simulink model "DCMotorControl"  (R2014a)
settings: Solver=ode45  StartTime=0.0  StopTime=10.0  RelTol=1e-3
InitFcn:
  | R = 8.70
  | Kt = 0.0334
  | Ke = 0.0334
  | J = 1.80e-6
  | L = 0
  | b = 0
settings Model: Creator=usmankhan  LastModifiedBy=usmankhan

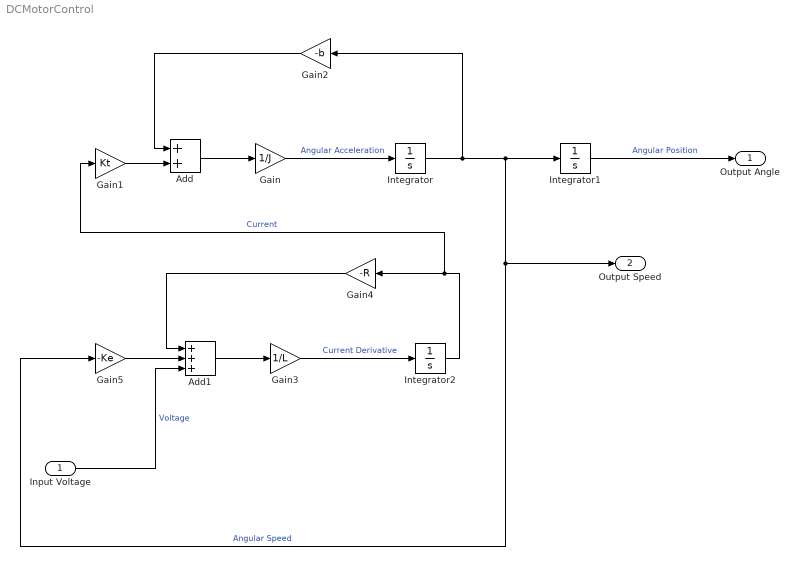
== system DCMotorControl ==
  Input Voltage : Inport
  Add : Sum
  Add1 : Sum  Inputs=+++
  Gain : Gain  Gain=1/J
  Gain1 : Gain  Gain=Kt
  Gain2 : Gain  Gain=-b
  Gain3 : Gain  Gain=1/L
  Gain4 : Gain  Gain=-R
  Gain5 : Gain  Gain=-Ke
  Integrator : Integrator
  Integrator1 : Integrator
  Integrator2 : Integrator
  Output Angle : Outport
  Output Speed : Outport  Port=2
  wires:
  Integrator1/1 -> Output Angle/1  "Angular Position"
  Gain/1 -> Integrator/1  "Angular Acceleration"
  Add/1 -> Gain/1
  Gain1/1 -> Add/2
  Gain2/1 -> Add/1
  Integrator2/1 -> Gain1/1, Gain4/1  "Current"
  Add1/1 -> Gain3/1
  Gain3/1 -> Integrator2/1  "Current Derivative"
  Gain4/1 -> Add1/1
  Gain5/1 -> Add1/2
  Input Voltage/1 -> Add1/3  "Voltage"
  Integrator/1 -> Gain2/1, Output Speed/1, Gain5/1, Integrator1/1  "Angular Speed"
